simulink model "simulate_fixed_drone"  (R2021a)
settings: Solver=VariableStepAuto  StartTime=0.0  StopTime=100  RelTol=1e-3
PreLoadFcn:
  | set_param_fixed;
undefined symbols (not defined in the file or in its folder): ParamFixLine, ParamFixOrb
settings Model: Creator=diogo  LastModifiedBy=Nunes
settings SolverCC: AlgebraicLoopSolver=TrustRegion
settings DebuggingCC: SFMachineParentedDataDiag=warning

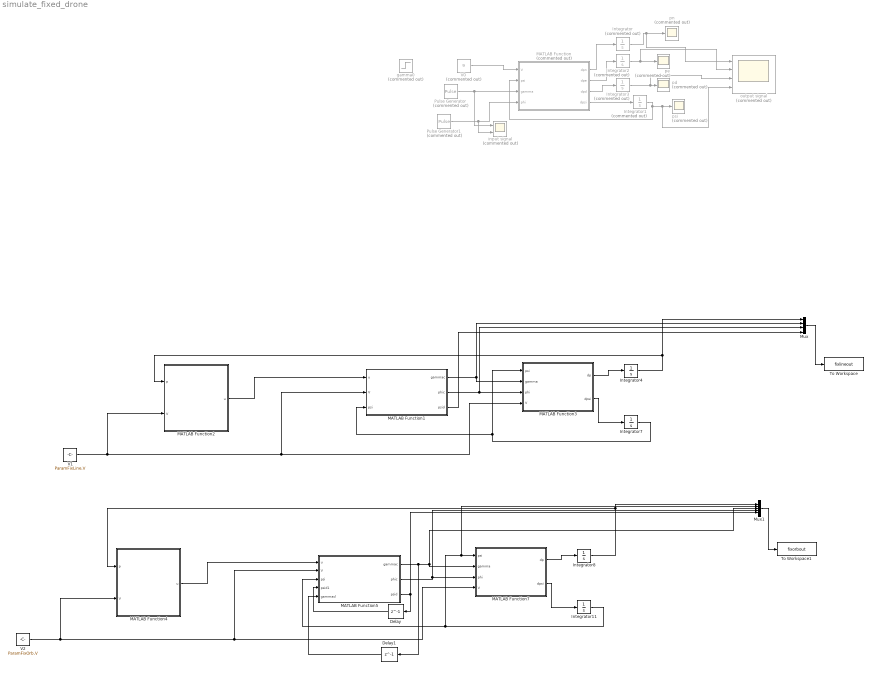
== system simulate_fixed_drone ==
  Delay : Delay  DelayLength=1  InitialCondition=0
  Delay1 : Delay  DelayLength=1  InitialCondition=0
  Integrator{,1..3} (4 alike) : Integrator  Commented=on
  Integrator11 : Integrator  InitialCondition=ParamFixOrb.psi0
  Integrator4 : Integrator  InitialCondition=ParamFixLine.p0
  Integrator7 : Integrator  InitialCondition=ParamFixLine.psi0
  Integrator8 : Integrator  InitialCondition=ParamFixOrb.p0
  MATLAB Function : MATLAB Function  Commented=on  TreatAsAtomicUnit=on
  MATLAB Function1 : MATLAB Function  TreatAsAtomicUnit=on
  MATLAB Function2 : MATLAB Function  TreatAsAtomicUnit=on
  MATLAB Function3 : MATLAB Function  TreatAsAtomicUnit=on
  MATLAB Function4 : MATLAB Function  TreatAsAtomicUnit=on
  MATLAB Function5 : MATLAB Function  TreatAsAtomicUnit=on
  MATLAB Function7 : MATLAB Function  TreatAsAtomicUnit=on
  Mux : Mux
  Mux1 : Mux  Inputs=5
  Pulse Generator : DiscretePulseGenerator  Commented=on  PulseType=Time based  Amplitude=0.087266  Period=20  PulseWidth=15  PhaseDelay=2
  Pulse Generator1 : DiscretePulseGenerator  Commented=on  PulseType=Time based  Amplitude=0.087266  Period=20  PulseWidth=15  PhaseDelay=13
  To Workspace : ToWorkspace  VariableName=fixlineout  SaveFormat=Timeseries  SampleTime=-1
  To Workspace1 : ToWorkspace  VariableName=fixorbout  SaveFormat=Timeseries  SampleTime=-1
  V0 : Constant  Commented=on  Value=9
  V1 : Constant  Value=ParamFixLine.V
  V2 : Constant  Value=ParamFixOrb.V
  gamma0 : Step  Commented=on  Time=5  After=0.087266  SampleTime=0
  input signal : Scope  Commented=on  NumInputPorts=2
  output signal : Scope  Commented=on  NumInputPorts=4
  pd : Scope  Commented=on
  pe : Scope  Commented=on
  pn : Scope  Commented=on
  psi : Scope  Commented=on
  wires:
  MATLAB Function/1(dpn) -> Integrator/1
  MATLAB Function/4(dpsi) -> Integrator1/1
  Integrator/1 -> output signal/1, pn/1
  Integrator1/1 -> output signal/4, psi/1, MATLAB Function/2(psi)
  V0/1 -> MATLAB Function/1(V)
  Pulse Generator1/1 -> input signal/2, MATLAB Function/4(phi)
  MATLAB Function/2(dpe) -> Integrator2/1
  MATLAB Function/3(dpd) -> Integrator3/1
  Integrator2/1 -> output signal/2, pe/1
  Integrator3/1 -> output signal/3, pd/1
  Pulse Generator/1 -> input signal/1, MATLAB Function/3(gamma)
  MATLAB Function3/1(dp) -> Integrator4/1
  MATLAB Function3/2(dpsi) -> Integrator7/1
  Integrator7/1 -> MATLAB Function1/3(psi), MATLAB Function3/1(psi)
  MATLAB Function1/2(phic) -> Mux/3, MATLAB Function3/3(phi)
  MATLAB Function1/1(gammac) -> MATLAB Function3/2(gamma), Mux/2
  V1/1 -> MATLAB Function2/2(V), MATLAB Function1/2(V), MATLAB Function3/4(V)
  Integrator4/1 -> MATLAB Function2/1(p), Mux/1
  MATLAB Function2/1(u) -> MATLAB Function1/1(u)
  Mux/1 -> To Workspace/1
  MATLAB Function5/2(phic) -> Mux1/4, MATLAB Function7/3(phi)
  MATLAB Function7/1(dp) -> Integrator8/1
  V2/1 -> MATLAB Function4/2(V), MATLAB Function5/2(V), MATLAB Function7/4(V)
  MATLAB Function7/2(dpsi) -> Integrator11/1
  Integrator11/1 -> Mux1/2, MATLAB Function7/1(psi), MATLAB Function5/3(psi)
  Mux1/1 -> To Workspace1/1
  MATLAB Function5/1(gammac) -> Delay1/1, Mux1/3, MATLAB Function7/2(gamma)
  Integrator8/1 -> MATLAB Function4/1(p), Mux1/1
  MATLAB Function4/1(u) -> MATLAB Function5/1(u)
  MATLAB Function5/3(psid) -> Mux1/5, Delay/1
  Delay/1 -> MATLAB Function5/4(psid1)
  MATLAB Function1/3(psid) -> Mux/4
  Delay1/1 -> MATLAB Function5/5(gammacl)

== matlab function simulate_fixed_drone/MATLAB Function1 ==
  data: u input; V input; psi input; gammac output; phic output; ParamFixLine parameter; psid output
function [  gammac, phic, psid] = path_following_controller(u, V, psi, ParamFixLine)


gamma_limit = ParamFixLine.gamma_limit;
phi_limit = ParamFixLine.phi_limit;
kphi = ParamFixLine.kphi;

gammac = -sat(asin(u(3)/V), gamma_limit);

psid = atan2(u(2),u(1));

phic = sat(kphi*(psid- psi), phi_limit);

end

== matlab function simulate_fixed_drone/MATLAB Function ==
  data: V input; dpn output; dpe output; dpd output; psi input; gamma input; phi input; dpsi output
function [dpn, dpe, dpd,dpsi] = drone_model(V,psi,gamma,phi)
    
    %criar param para generalizar os valores
    
    %dp = [V*cos(psi)*cos(gamma); V*sin(psi)*cos(gamma); -V*sin(gamma)]
    
    dpn =V*cos(psi)*cos(gamma);
    dpe = V*sin(psi)*cos(gamma);
    dpd = -V*sin(gamma);
    dpsi =  (9.8/V)*tan(phi);
    
    
end

== matlab function simulate_fixed_drone/MATLAB Function2 ==
  data: p input; u output; V input; ParamFixLine parameter
function u  = straight_path_generator(p, V, ParamFixLine)


%Variables

psi_l = ParamFixLine.psi_l;  %desired heading angle
gamma_l = ParamFixLine.gamma_l; %desired flight path angle

c_n = ParamFixLine.c0(1);    %path starting point
c_e = ParamFixLine.c0(2);
c_d = ParamFixLine.c0(3);

r_n = p(1);    %position
r_e = p(2);
r_d = p(3);
r = [r_n; r_e; r_d];

cl = [c_n; c_e; c_d];

ql = [cos(psi_l)*cos(gamma_l) ; sin(psi_l)*cos(gamma_l) ; -sin(gamma_l) ];
%direction of line




n_lon = [ -sin(psi_l) ; cos(psi_l) ; 0 ]; 

n_lat = [-cos(psi_l)*sin(gamma_l) ; -sin(psi_l)*sin(gamma_l) ; -cos(gamma_l) ];

k1 = 1;
k2 = 10;

%u_line = k1*(n_lon*transpose(n_lon) +  n_lat*transpose(n_lat))*(r - cl) + k2*cross(n_lon,n_lat);
u_line = -k1*(n_lon*n_lon' +  n_lat*n_lat')*(r - cl) - k2*cross(n_lon,n_lat);

u = V*(u_line/norm(u_line));



end

== matlab function simulate_fixed_drone/MATLAB Function3 ==
  data: psi input; gamma input; phi input; V input; dp output; dpsi output
function [dp, dpsi] = drone_model(psi,gamma,phi, V)
    
    %criar param para generalizar os valores
    
    %dp = [V*cos(psi)*cos(gamma); V*sin(psi)*cos(gamma); -V*sin(gamma)]
    
    dpn =V*cos(psi)*cos(gamma);
    dpe = V*sin(psi)*cos(gamma);
    dpd = -V*sin(gamma);
    dpsi =  (9.8/V)*tan(phi);
    
    dp = [dpn; dpe; dpd];
end

== matlab function simulate_fixed_drone/MATLAB Function4 ==
  data: p input; u output; V input; ParamFixOrb parameter
function u  = orbit_path_generator(p, V, ParamFixOrb)


%Variables

 Rh = ParamFixOrb.Rh;
 lambda = ParamFixOrb.lambda;
 gamma_h = ParamFixOrb.gamma_h;
 psi_h = ParamFixOrb.psi_h;
 
k1 = ParamFixOrb.k1;
k2 = ParamFixOrb.k2;
 

ch = ParamFixOrb.ch;

c_n = ch(1);    %center of helix
c_e = ch(2);
c_d = ch(3);


 r_n = p(1);
 r_e = p(2);
 r_d = p(3);
 
 
%r0 = ch + [Rh*cos(psi_h) ; Rh*sin(psi_h) ; 0];

dalpha_cyl = transpose( [ 2*(r_n - c_n)/Rh ; 2*(r_e - c_e)/Rh ; 0 ] );

dalpha_pl = transpose( [ (tan(gamma_h)/lambda)*(-(r_e - c_e))/( (r_n - c_n)^2 + (r_e - c_e)^2 ) ; (tan(gamma_h)/lambda)*(r_n - c_n)/( (r_n - c_n)^2 + (r_e - c_e)^2 )  ; 1/Rh ] );


alpha_cyl = ( (r_n - c_n)/Rh )^2 + ( (r_e - c_e)/Rh )^2 -1;

alpha_pl = ( (r_d - c_d)/Rh )^2 + (tan(gamma_h)/lambda)*(atan( (r_e - c_e)/(r_n - c_n) ) - psi_h);

u_line = k1*(-alpha_cyl*dalpha_cyl - alpha_pl*dalpha_pl) - lambda*k2*( (2/Rh)*transpose([ (r_e - c_e)/Rh ; -(r_n - c_n)/Rh ; lambda*tan(gamma_h) ]) );

u =  V*(u_line/norm(u_line));





end

== matlab function simulate_fixed_drone/MATLAB Function5 ==
  data: u input; V input; psi input; psid1 input; gammacl input; gammac output; phic output; ParamFixOrb parameter; psid output
function [  gammac, phic, psid] = path_following_controller(u, V, psi, psid1, gammacl, ParamFixOrb)

gamma_limit = ParamFixOrb.gamma_limit;
phi_limit = ParamFixOrb.phi_limit;
kphi = ParamFixOrb.kphi;

gammac = -sat(asin(u(3)/V), gamma_limit);


% while abs(gammac - gammacl) > 3*pi/2
%     if((gammac - gammacl) > 3*pi/2) 
%         gammac = gammacl- 2*pi;
%     elseif ((gammac - gammacl) < - 3*pi/2)
%         gammac = gammac + 2*pi;
%     end
% end



psid = atan2(u(2),u(1));

while abs(psid - psid1) > 3*pi/2
    if((psid - psid1) > 3*pi/2) 
        psid = psid- 2*pi;
    elseif ((psid - psid1) < - 3*pi/2)
        psid = psid + 2*pi;
    end
end

if(abs(psid - psid1) > pi)
    xpto = 0;
end;

phic = sat(kphi*(psid - psi), phi_limit);

end

== matlab function simulate_fixed_drone/MATLAB Function7 ==
  data: psi input; gamma input; phi input; V input; dp output; dpsi output
function [dp,dpsi] = drone_model(psi,gamma,phi, V)
    
    %criar param para generalizar os valores
    
    %dp = [V*cos(psi)*cos(gamma); V*sin(psi)*cos(gamma); -V*sin(gamma)]
    
    dpn =V*cos(psi)*cos(gamma);
    dpe = V*sin(psi)*cos(gamma);
    dpd = -V*sin(gamma);
    dpsi =  (9.8/V)*tan(phi);
    
    dp = [dpn; dpe; dpd];
    
end
